simulink model "push_pull"  (R2018a)
settings: Solver=VariableStepAuto  StartTime=0.0  StopTime=0.05  RelTol=1e-3
libraries: powerlib x13
settings Model: Creator=burya  LastModifiedBy=burya

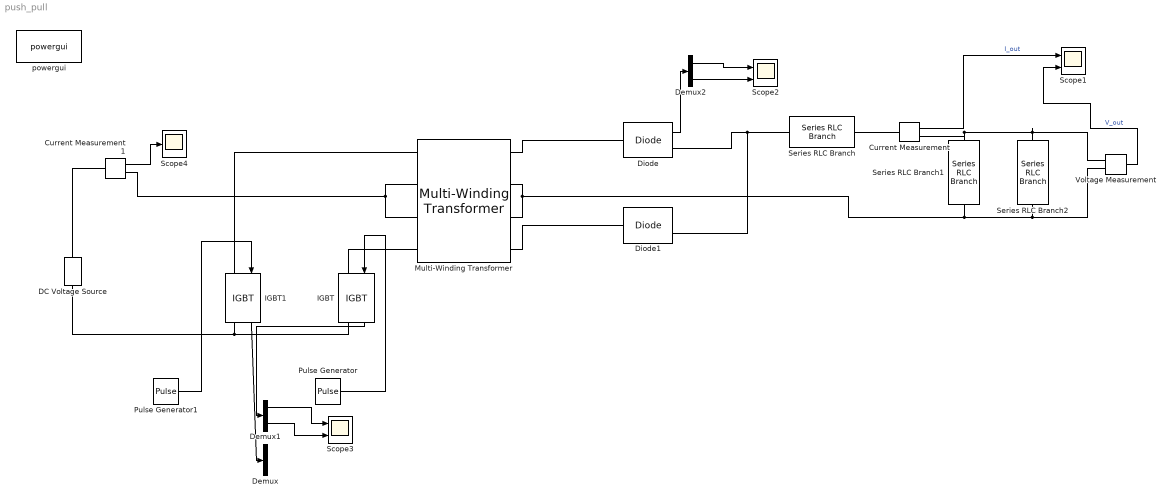
== system push_pull ==
  Current Measurement : powerlib/Measurements/Current Measurement  PhasorSimulation=off  OutputType=Complex  PSBequivalent=0
  Current Measurement1 : powerlib/Measurements/Current Measurement  PhasorSimulation=off  OutputType=Complex  PSBequivalent=0
  DC Voltage Source : powerlib/Electrical Sources/DC Voltage Source  Amplitude=48  Measurements=None
  Demux : Demux  Outputs=2
  Demux1 : Demux  Outputs=2
  Demux2 : Demux  Outputs=2
  Diode : powerlib/Power Electronics/Diode  Ron=0.001  Lon=0  Vf=0  IC=0  UseSnubber=0  Rs=inf  Cs=250e-9  Measurements=on
  Diode1 : powerlib/Power Electronics/Diode  Ron=0.001  Lon=0  Vf=0  IC=0  UseSnubber=0  Rs=inf  Cs=250e-9  Measurements=on
  IGBT : powerlib/Power Electronics/IGBT  Ron=0.001  Lon=0  Vf=1  Tf=1e-6  Tt=2e-6  IC=0  Rs=1e5  Cs=inf  Measurements=on
  IGBT1 : powerlib/Power Electronics/IGBT  Ron=0.001  Lon=0  Vf=1  Tf=1e-6  Tt=2e-6  IC=0  Rs=1e5  Cs=inf  Measurements=on
  Multi-Winding Transformer : powerlib/Elements/Multi-Winding Transformer  LeftWindings=2  RightWindings=2  TappedWindings=no taps  NumberOfTaps=1  SetSaturation=off  Hysteresis=off  DataFile='hysteresis.mat'  Measurements=None  UNITS=SI  NominalPower=[96 40e3]  NominalVoltages=[48 48 24 24 ]  WindingResistances=[29e-3 29e-3 4e-3 4e-3]  WindingInductances=[0 0 0 0]  Rm=3.8221e+9  Lm=0.74e-3  Saturation=[0 0;0.13021 3501.7;54.254 4435.4]  MoreParameters=off  BreakLoop=off  DataType=on  InitialFlux=0  TransfoNumber=1
      settings: SourceProductName=Simscape Power Systems  SourceProductBaseCode=PS
  Pulse Generator : DiscretePulseGenerator  PulseType=Time based  Period=1/40e3  PulseWidth=25
  Pulse Generator1 : DiscretePulseGenerator  PulseType=Time based  Period=1/40e3  PulseWidth=25  PhaseDelay=1/80e3
  Scope1 : Scope  NumInputPorts=2
  Scope2 : Scope  NumInputPorts=2
  Scope3 : Scope  NumInputPorts=2
  Scope4 : Scope
  Series RLC Branch : powerlib/Elements/Series RLC Branch  LConnTagsString=__new0  RConnTagsString=__new0  BranchType=RL  Resistance=13.9e-3  Inductance=0.55e-3  SetiL0=off  InitialCurrent=0  Capacitance=1e-6  Setx0=off  InitialVoltage=0  Measurements=None
  Series RLC Branch1 : powerlib/Elements/Series RLC Branch  LConnTagsString=__new0  RConnTagsString=__new0  BranchType=C  Resistance=1  Inductance=0.55e-3  SetiL0=off  InitialCurrent=0  Capacitance=30e-6  Setx0=off  InitialVoltage=0  Measurements=None
  Series RLC Branch2 : powerlib/Elements/Series RLC Branch  LConnTagsString=__new0  RConnTagsString=__new0  BranchType=R  Resistance=12/8  Inductance=0.55e-3  SetiL0=off  InitialCurrent=0  Capacitance=30e-6  Setx0=off  InitialVoltage=0  Measurements=None
  Voltage Measurement : powerlib/Measurements/Voltage Measurement  PhasorSimulation=off  OutputType=Complex  PSBequivalent=0
  powergui : powerlib/powergui  Priority=1  SimulationMode=Continuous  SampleTime=50e-6  frequency=60  Iterations=50  frequencyindice=0  Pbase=100e6  ErrMax=1e-4  UnitsV=kV  UnitsW=MW  buscounter=0  FunctionMessages=off  echomessages=off  EnableUseOfTLC=off  CurrentSourceSwitches=off  DisableSnubberDevices=off  DisableRonSwitches=off  DisableVfSwitches=off  DisplayEquations=off  SolverType=Tustin/Backward Euler (TBE)  Interpol=off  ExternalGateDelay=off  methode=off  Ts=100  x0status=blocks  SPID=on  SwTol=0  HookPort=off  RestoreLinks=warning  ResistiveCurrentMeasurement=off  Frange=[0:2:500]  Ylog=off  Xlog=on  ShowGrid=off  save=off  variable=ZData  structure=0  ZoomFFT=off  StartTime=0.0  cycles=1  DisplayStyle=1  fundamental=60  FreqAxis=off  MaxFrequency=1000  frequencyindicesteady=1  RmsSteady=1  display=off
  wires:
  Pulse Generator/1 -> IGBT/1
  Pulse Generator1/1 -> IGBT1/1
  IGBT1/1 -> Demux/1
  IGBT/1 -> Demux1/1
  Voltage Measurement/1 -> Scope1/2  "V_out"
  Current Measurement/1 -> Scope1/1  "I_out"
  Current Measurement1/1 -> Scope4/1
  Demux1/1 -> Scope3/1
  Demux1/2 -> Scope3/2
  Demux2/1 -> Scope2/1
  Demux2/2 -> Scope2/2
  Diode/1 -> Demux2/1
  connections:
  Multi-Winding Transformer/LConn3 -- Multi-Winding Transformer/LConn2 -- Current Measurement1/RConn1
  DC Voltage Source/LConn1 -- IGBT1/RConn1 -- IGBT/RConn1
  IGBT1/LConn1 -- Multi-Winding Transformer/LConn1
  IGBT/LConn1 -- Multi-Winding Transformer/LConn4
  Diode/LConn1 -- Multi-Winding Transformer/RConn1
  Diode/RConn1 -- Diode1/RConn1 -- Series RLC Branch/LConn1
  Series RLC Branch2/LConn1 -- Voltage Measurement/LConn1 -- Current Measurement/RConn1 -- Series RLC Branch1/LConn1
  Current Measurement/LConn1 -- Series RLC Branch/RConn1
  Current Measurement1/LConn1 -- DC Voltage Source/RConn1
  Diode1/LConn1 -- Multi-Winding Transformer/RConn4
  Series RLC Branch1/RConn1 -- Multi-Winding Transformer/RConn2 -- Multi-Winding Transformer/RConn3 -- Voltage Measurement/LConn2 -- Series RLC Branch2/RConn1
